simulink model "SimNL_Subsystems"  (R2016b)
settings: Solver=VariableStepAuto  StartTime=0.0  StopTime=10  FixedStep=SampleTime  RelTol=1e-3
values from neighbouring files (symbols this model uses):
  AC = []    [SetupNL.m]
undefined symbols (not defined in the file or in its folder): Env, Sim
libraries: OpenFlightUtilLib x17, SimCoreLib x3
(part 2 of 2)

== system SimNL_Subsystems/SubSystemModels/Aero_VarGen/AeroCoefLookup/PitchMomentCoefficient ==
  TableDep : Inport
  StabDep : Inport  Port=2
  CntrlDep : Inport  Port=3
  Bus Selector1 : BusSelector  OutputSignals=vTrue_mps,alpha_rad,beta_rad
  Bus Selector4 : BusSelector  OutputSignals=vTrue_mps,alpha_rad,beta_rad
  Constant1 : Constant  Value=AC.Aero.Cm.tableSelCntrl
      settings: AttributesFormatString=%<Value>
  Constant2 : Constant  Value=AC.Aero.Cm.tableSelStab
      settings: AttributesFormatString=%<Value>
  Dot Product : DotProduct  InputSameDT=on  OutDataTypeStr=Inherit: Inherit via internal rule
  Dot Product1 : DotProduct  InputSameDT=on  OutDataTypeStr=Inherit: Inherit via internal rule
  Sum : Sum  Inputs=|++
  n-D Lookup Table : Lookup_n-D  NumberOfTableDimensions=AC.Aero.tableDim  BreakpointsForDimension1=AC.Aero.breakPts{1}  BreakpointsForDimension2=AC.Aero.breakPts{2}  BreakpointsForDimension3=AC.Aero.breakPts{3}  BreakpointsForDimension4=AC.Aero.Cm.tableSelStab  Table=AC.Aero.Cm.tableStab  InternalRulePriority=Speed  RndMeth=Simplest  InputSameDT=on
      settings: AttributesFormatString=%<Table>
  n-D Lookup Table1 : Lookup_n-D  NumberOfTableDimensions=AC.Aero.tableDim  BreakpointsForDimension1=AC.Aero.breakPts{1}  BreakpointsForDimension2=AC.Aero.breakPts{2}  BreakpointsForDimension3=AC.Aero.breakPts{3}  BreakpointsForDimension4=AC.Aero.Cm.tableSelCntrl  Table=AC.Aero.Cm.tableCntrl  InternalRulePriority=Speed  RndMeth=Simplest  InputSameDT=on
      settings: AttributesFormatString=%<Table>
  Cm : Outport
  wires:
  Dot Product/1 -> Sum/1
  Constant2/1 -> n-D Lookup Table/4
  n-D Lookup Table/1 -> Dot Product/1  "Cm_Stab"
  StabDep/1 -> Dot Product/2
  TableDep/1 -> Bus Selector1/1, Bus Selector4/1
  Constant1/1 -> n-D Lookup Table1/4
  CntrlDep/1 -> Dot Product1/2
  n-D Lookup Table1/1 -> Dot Product1/1  "Cm_Cntrl"
  Dot Product1/1 -> Sum/2
  Sum/1 -> Cm/1  "Cm"
  Bus Selector1/1 -> n-D Lookup Table1/1  "<vTrue_mps>"
  Bus Selector1/3 -> n-D Lookup Table1/3  "<beta_rad>"
  Bus Selector1/2 -> n-D Lookup Table1/2  "<alpha_rad>"
  Bus Selector4/3 -> n-D Lookup Table/3  "<beta_rad>"
  Bus Selector4/2 -> n-D Lookup Table/2  "<alpha_rad>"
  Bus Selector4/1 -> n-D Lookup Table/1  "<vTrue_mps>"

== system SimNL_Subsystems/SubSystemModels/Aero_VarGen/AeroCoefLookup/RollMomentCoefficient ==
  TableDep : Inport
  StabDep : Inport  Port=2
  CntrlDep : Inport  Port=3
  Bus Selector1 : BusSelector  OutputSignals=vTrue_mps,alpha_rad,beta_rad
  Bus Selector4 : BusSelector  OutputSignals=vTrue_mps,alpha_rad,beta_rad
  Constant1 : Constant  Value=AC.Aero.Cl.tableSelCntrl
      settings: AttributesFormatString=%<Value>
  Constant2 : Constant  Value=AC.Aero.Cl.tableSelStab
      settings: AttributesFormatString=%<Value>
  Dot Product : DotProduct  InputSameDT=on  OutDataTypeStr=Inherit: Inherit via internal rule
  Dot Product1 : DotProduct  InputSameDT=on  OutDataTypeStr=Inherit: Inherit via internal rule
  Sum : Sum  Inputs=|++
  n-D Lookup Table : Lookup_n-D  NumberOfTableDimensions=AC.Aero.tableDim  BreakpointsForDimension1=AC.Aero.breakPts{1}  BreakpointsForDimension2=AC.Aero.breakPts{2}  BreakpointsForDimension3=AC.Aero.breakPts{3}  BreakpointsForDimension4=AC.Aero.Cl.tableSelStab  Table=AC.Aero.Cl.tableStab  InternalRulePriority=Speed  RndMeth=Simplest  InputSameDT=on
      settings: AttributesFormatString=%<Table>
  n-D Lookup Table1 : Lookup_n-D  NumberOfTableDimensions=AC.Aero.tableDim  BreakpointsForDimension1=AC.Aero.breakPts{1}  BreakpointsForDimension2=AC.Aero.breakPts{2}  BreakpointsForDimension3=AC.Aero.breakPts{3}  BreakpointsForDimension4=AC.Aero.Cl.tableSelCntrl  Table=AC.Aero.Cl.tableCntrl  InternalRulePriority=Speed  RndMeth=Simplest  InputSameDT=on
      settings: AttributesFormatString=%<Table>
  Cl : Outport
  wires:
  Dot Product/1 -> Sum/1
  Constant2/1 -> n-D Lookup Table/4
  n-D Lookup Table/1 -> Dot Product/1  "Cl_Stab"
  StabDep/1 -> Dot Product/2
  TableDep/1 -> Bus Selector1/1, Bus Selector4/1
  Constant1/1 -> n-D Lookup Table1/4
  CntrlDep/1 -> Dot Product1/2
  n-D Lookup Table1/1 -> Dot Product1/1  "Cl_Cntrl"
  Dot Product1/1 -> Sum/2
  Sum/1 -> Cl/1  "Cl"
  Bus Selector4/1 -> n-D Lookup Table/1  "<vTrue_mps>"
  Bus Selector4/2 -> n-D Lookup Table/2  "<alpha_rad>"
  Bus Selector4/3 -> n-D Lookup Table/3  "<beta_rad>"
  Bus Selector1/1 -> n-D Lookup Table1/1  "<vTrue_mps>"
  Bus Selector1/2 -> n-D Lookup Table1/2  "<alpha_rad>"
  Bus Selector1/3 -> n-D Lookup Table1/3  "<beta_rad>"

== system SimNL_Subsystems/SubSystemModels/Aero_VarGen/AeroCoefLookup/SideForceCoefficient ==
  TableDep : Inport
  StabDep : Inport  Port=2
  CntrlDep : Inport  Port=3
  Bus Selector1 : BusSelector  OutputSignals=vTrue_mps,alpha_rad,beta_rad
  Bus Selector4 : BusSelector  OutputSignals=vTrue_mps,alpha_rad,beta_rad
  Constant1 : Constant  Value=AC.Aero.CY.tableSelCntrl
      settings: AttributesFormatString=%<Value>
  Constant2 : Constant  Value=AC.Aero.CY.tableSelStab
      settings: AttributesFormatString=%<Value>
  Dot Product : DotProduct  InputSameDT=on  OutDataTypeStr=Inherit: Inherit via internal rule
  Dot Product1 : DotProduct  InputSameDT=on  OutDataTypeStr=Inherit: Inherit via internal rule
  Sum : Sum  Inputs=|++
  n-D Lookup Table : Lookup_n-D  NumberOfTableDimensions=AC.Aero.tableDim  BreakpointsForDimension1=AC.Aero.breakPts{1}  BreakpointsForDimension2=AC.Aero.breakPts{2}  BreakpointsForDimension3=AC.Aero.breakPts{3}  BreakpointsForDimension4=AC.Aero.CY.tableSelStab  Table=AC.Aero.CY.tableStab  InternalRulePriority=Speed  RndMeth=Simplest  InputSameDT=on
      settings: AttributesFormatString=%<Table>
  n-D Lookup Table1 : Lookup_n-D  NumberOfTableDimensions=AC.Aero.tableDim  BreakpointsForDimension1=AC.Aero.breakPts{1}  BreakpointsForDimension2=AC.Aero.breakPts{2}  BreakpointsForDimension3=AC.Aero.breakPts{3}  BreakpointsForDimension4=AC.Aero.CY.tableSelCntrl  Table=AC.Aero.CY.tableCntrl  InternalRulePriority=Speed  RndMeth=Simplest  InputSameDT=on
      settings: AttributesFormatString=%<Table>
  CY : Outport
  wires:
  Dot Product/1 -> Sum/1
  Bus Selector4/1 -> n-D Lookup Table/1  "<vTrue_mps>"
  Bus Selector4/2 -> n-D Lookup Table/2  "<alpha_rad>"
  Constant2/1 -> n-D Lookup Table/4
  n-D Lookup Table/1 -> Dot Product/1  "CY_Stab"
  StabDep/1 -> Dot Product/2
  TableDep/1 -> Bus Selector1/1, Bus Selector4/1
  Constant1/1 -> n-D Lookup Table1/4
  CntrlDep/1 -> Dot Product1/2
  n-D Lookup Table1/1 -> Dot Product1/1  "CY_Cntrl"
  Dot Product1/1 -> Sum/2
  Sum/1 -> CY/1  "CY"
  Bus Selector4/3 -> n-D Lookup Table/3  "<beta_rad>"
  Bus Selector1/1 -> n-D Lookup Table1/1  "<vTrue_mps>"
  Bus Selector1/2 -> n-D Lookup Table1/2  "<alpha_rad>"
  Bus Selector1/3 -> n-D Lookup Table1/3  "<beta_rad>"

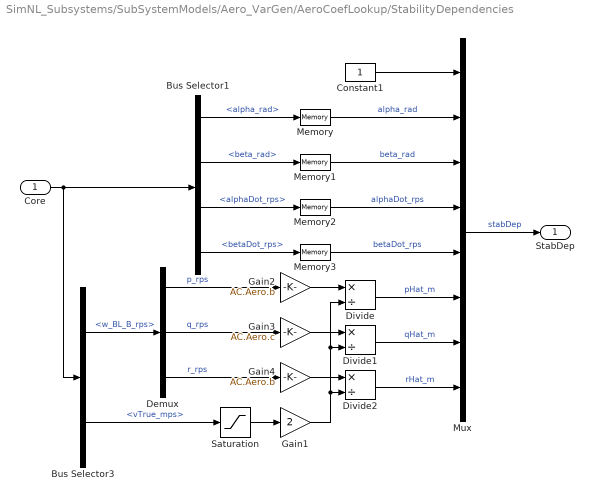
== system SimNL_Subsystems/SubSystemModels/Aero_VarGen/AeroCoefLookup/StabilityDependencies ==
  Core : Inport
  Bus Selector1 : BusSelector  OutputSignals=BusAux.BusFlow.alpha_rad,BusAux.BusFlow.beta_rad,BusAux.BusFlow.alphaDot_rps,BusAux.BusFlow.betaDot_rps
  Bus Selector3 : BusSelector  OutputSignals=BusEom.w_BL_B_rps,BusAux.BusFlow.vTrue_mps
  Constant1 : Constant
  Demux : Demux  Outputs=3
  Divide : Product  Inputs=*/
  Divide1 : Product  Inputs=*/
  Divide2 : Product  Inputs=*/
  Gain1 : Gain  Gain=2  SaturateOnIntegerOverflow=on  OutDataTypeStr=Inherit: Same as input  ParamDataTypeStr=Inherit: Same as input
  Gain2 : Gain  Gain=AC.Aero.b  SaturateOnIntegerOverflow=on  OutDataTypeStr=Inherit: Same as input  ParamDataTypeStr=Inherit: Same as input
      settings: AttributesFormatString=%<Gain>
  Gain3 : Gain  Gain=AC.Aero.c  SaturateOnIntegerOverflow=on  OutDataTypeStr=Inherit: Same as input  ParamDataTypeStr=Inherit: Same as input
      settings: AttributesFormatString=%<Gain>
  Gain4 : Gain  Gain=AC.Aero.b  SaturateOnIntegerOverflow=on  OutDataTypeStr=Inherit: Same as input  ParamDataTypeStr=Inherit: Same as input
      settings: AttributesFormatString=%<Gain>
  Memory : Memory  X0=Sim.Trim.Init.alpha_rad  InheritSampleTime=on  LinearizeMemory=on  StateIdentifier=alphaState_rad
      settings: AttributesFormatString=%<StateIdentifier>
  Memory1 : Memory  X0=Sim.Trim.Init.beta_rad  InheritSampleTime=on  LinearizeMemory=on  StateIdentifier=betaState_rad
      settings: AttributesFormatString=%<StateIdentifier>
  Memory2 : Memory  X0=Sim.Trim.Init.alphaDot_rps  InheritSampleTime=on  LinearizeMemory=on  StateIdentifier=alphaDotState_rps
      settings: AttributesFormatString=%<StateIdentifier>
  Memory3 : Memory  X0=Sim.Trim.Init.betaDot_rps  InheritSampleTime=on  LinearizeMemory=on  StateIdentifier=betaDotState_rps
      settings: AttributesFormatString=%<StateIdentifier>
  Mux : Mux  Inputs=length(AC.Aero.CL.tableSelStab)
  Saturation : Saturate  UpperLimit=inf  LowerLimit=0.1
  StabDep : Outport
  wires:
  Bus Selector1/3 -> Memory2/1  "<alphaDot_rps>"
  Divide/1 -> Mux/6  "pHat_m"
  Bus Selector1/2 -> Memory1/1  "<beta_rad>"
  Bus Selector1/4 -> Memory3/1  "<betaDot_rps>"
  Core/1 -> Bus Selector3/1, Bus Selector1/1
  Constant1/1 -> Mux/1
  Mux/1 -> StabDep/1  "stabDep"
  Bus Selector1/1 -> Memory/1  "<alpha_rad>"
  Gain2/1 -> Divide/1
  Gain1/1 -> Divide1/2, Divide/2, Divide2/2
  Divide1/1 -> Mux/7  "qHat_m"
  Divide2/1 -> Mux/8  "rHat_m"
  Gain3/1 -> Divide1/1
  Gain4/1 -> Divide2/1
  Bus Selector3/2 -> Saturation/1  "<vTrue_mps>"
  Saturation/1 -> Gain1/1
  Bus Selector3/1 -> Demux/1  "<w_BL_B_rps>"
  Demux/1 -> Gain2/1  "p_rps"
  Demux/2 -> Gain3/1  "q_rps"
  Demux/3 -> Gain4/1  "r_rps"
  Memory/1 -> Mux/2  "alpha_rad"
  Memory1/1 -> Mux/3  "beta_rad"
  Memory2/1 -> Mux/4  "alphaDot_rps"
  Memory3/1 -> Mux/5  "betaDot_rps"

== system SimNL_Subsystems/SubSystemModels/Aero_VarGen/AeroCoefLookup/TableDependencies ==
  Core : Inport
  Bus Creator : BusCreator  Inputs=3
  Bus Selector4 : BusSelector  OutputSignals=BusAux.BusFlow.vTrue_mps,BusAux.BusFlow.alpha_rad,BusAux.BusFlow.beta_rad
  TableDep : Outport
  wires:
  Core/1 -> Bus Selector4/1
  Bus Selector4/1 -> Bus Creator/1  "<vTrue_mps>"
  Bus Selector4/3 -> Bus Creator/3  "<beta_rad>"
  Bus Selector4/2 -> Bus Creator/2  "<alpha_rad>"
  Bus Creator/1 -> TableDep/1  "tableDep"

== system SimNL_Subsystems/SubSystemModels/Aero_VarGen/AeroCoefLookup/YawMomentCoefficient ==
  TableDep : Inport
  StabDep : Inport  Port=2
  CntrlDep : Inport  Port=3
  Bus Selector1 : BusSelector  OutputSignals=vTrue_mps,alpha_rad,beta_rad
  Bus Selector4 : BusSelector  OutputSignals=vTrue_mps,alpha_rad,beta_rad
  Constant1 : Constant  Value=AC.Aero.Cn.tableSelCntrl
      settings: AttributesFormatString=%<Value>
  Constant2 : Constant  Value=AC.Aero.Cn.tableSelStab
      settings: AttributesFormatString=%<Value>
  Dot Product : DotProduct  InputSameDT=on  OutDataTypeStr=Inherit: Inherit via internal rule
  Dot Product1 : DotProduct  InputSameDT=on  OutDataTypeStr=Inherit: Inherit via internal rule
  Sum : Sum  Inputs=|++
  n-D Lookup Table : Lookup_n-D  NumberOfTableDimensions=AC.Aero.tableDim  BreakpointsForDimension1=AC.Aero.breakPts{1}  BreakpointsForDimension2=AC.Aero.breakPts{2}  BreakpointsForDimension3=AC.Aero.breakPts{3}  BreakpointsForDimension4=AC.Aero.Cn.tableSelStab  Table=AC.Aero.Cn.tableStab  InternalRulePriority=Speed  RndMeth=Simplest  InputSameDT=on
      settings: AttributesFormatString=%<Table>
  n-D Lookup Table1 : Lookup_n-D  NumberOfTableDimensions=AC.Aero.tableDim  BreakpointsForDimension1=AC.Aero.breakPts{1}  BreakpointsForDimension2=AC.Aero.breakPts{2}  BreakpointsForDimension3=AC.Aero.breakPts{3}  BreakpointsForDimension4=AC.Aero.Cn.tableSelCntrl  Table=AC.Aero.Cn.tableCntrl  InternalRulePriority=Speed  RndMeth=Simplest  InputSameDT=on
      settings: AttributesFormatString=%<Table>
  Cn : Outport
  wires:
  Dot Product/1 -> Sum/1
  Constant2/1 -> n-D Lookup Table/4
  n-D Lookup Table/1 -> Dot Product/1  "Cn_Stab"
  StabDep/1 -> Dot Product/2
  TableDep/1 -> Bus Selector1/1, Bus Selector4/1
  Constant1/1 -> n-D Lookup Table1/4
  CntrlDep/1 -> Dot Product1/2
  n-D Lookup Table1/1 -> Dot Product1/1  "Cn_Cntrl"
  Dot Product1/1 -> Sum/2
  Sum/1 -> Cn/1  "Cn"
  Bus Selector1/1 -> n-D Lookup Table1/1  "<vTrue_mps>"
  Bus Selector1/2 -> n-D Lookup Table1/2  "<alpha_rad>"
  Bus Selector1/3 -> n-D Lookup Table1/3  "<beta_rad>"
  Bus Selector4/1 -> n-D Lookup Table/1  "<vTrue_mps>"
  Bus Selector4/2 -> n-D Lookup Table/2  "<alpha_rad>"
  Bus Selector4/3 -> n-D Lookup Table/3  "<beta_rad>"
